simulink model "BBC_10"  (R2022b)
settings: Solver=VariableStepAuto  StartTime=0.0  StopTime=1.5  RelTol=1e-3
undefined symbols (not defined in the file): dEv, sigbuilder_block, X, Y
libraries: spsMosfetLib x4, spsSeriesRLCBranchLib x4, spsCurrentMeasurementLib x2, spsVoltageMeasurementLib x2, dspstat3 x1, simulink x1, spsGroundLib x1, spsControlledVoltageSourceLib x1, spspowerguiLib x1
settings Model: Creator=Dopechuro  LastModifiedBy=Dopechuro

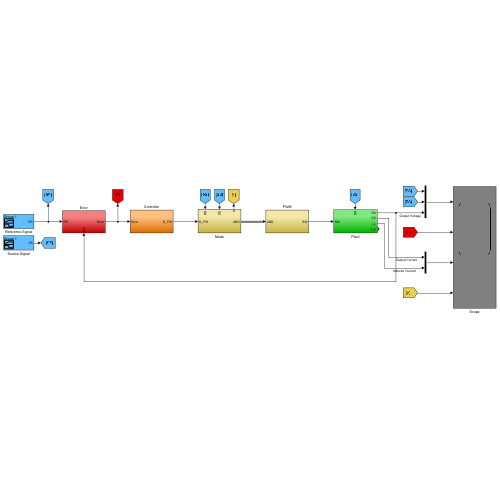
[thumbnail: Simulink's stored preview of the top-level diagram]
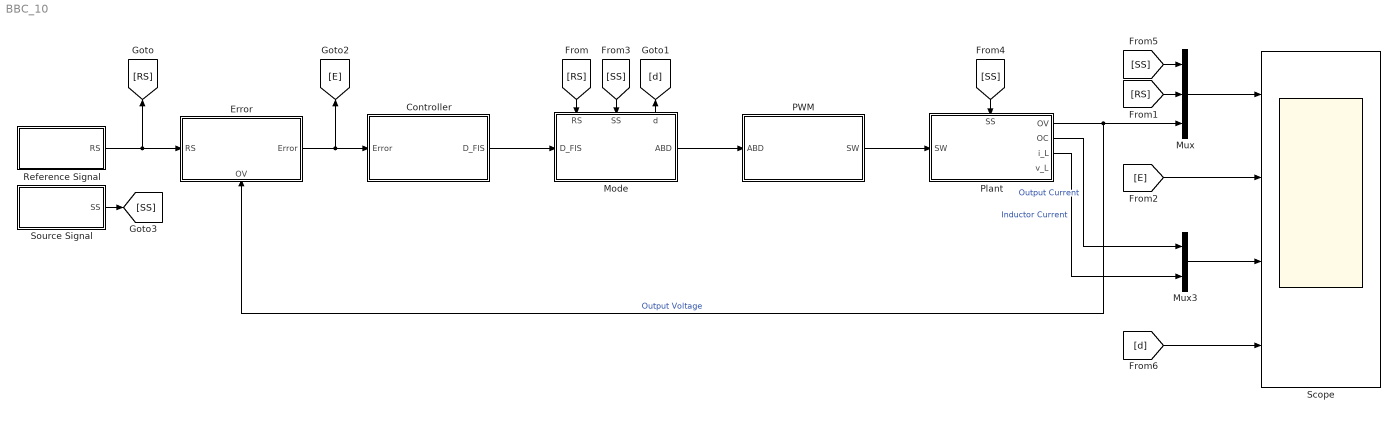
== system BBC_10 ==
  Controller : Subsystem
  Error : Subsystem
      settings: PortSchema="{\"entries\":[{\"content\":{\"sides\":[{\"content\":{\"connectorIds\":[\"In1\"]},\"type\":\"ConnectorPlacement.EquallySpacedRectSide\",\"uuid\":\"17a1441e-cc20-45c1-b94d-2797150f41f6\"},{\"content\":{\"connectorIds\":[\"Out1\"],\"side\":\"RIGHT\"},\"type\":\"ConnectorPlacement.EquallySpacedRectSide\",\"uuid\":\"0eaf207d-efc8-435f-a7b8-030690917f23\"},{\"content\":{\"connectorIds\":[],\"side\":\"TOP\"},\"type\":\"ConnectorPlacement.EquallySpacedRectSide\",\"uuid\":\"e36a2cea-826c-4841-9b9b-81d458cfbbc3\"},{\"content\":{\"connectorIds\":[\"In2\"],\"side\":\"BOTTOM\"},\"type\":\"ConnectorPlacement.EquallySpacedRectSide\",\"uuid\":\"071bf484-cc76-4d4d-9853-4ed74954b615\"}]},\"type\":\"ConnectorPlacement.EquallySpacedConnector\",\"uuid\":\"670cfee0-0ffb-439b-ae3a-e57aa259e987\"}],\"packageUris\":[\"http://schema.mathworks.com/mf0/Connector/R2020b\"],\"version\":\"1.0\"}"
  Mode : Subsystem
      settings: PortSchema="{\"entries\":[{\"content\":{\"sides\":[{\"content\":{\"connectorIds\":[\"In1\"]},\"type\":\"ConnectorPlacement.EquallySpacedRectSide\",\"uuid\":\"22e8c9bf-f581-4102-833a-b5611cc3792f\"},{\"content\":{\"connectorIds\":[\"Out1\"],\"side\":\"RIGHT\"},\"type\":\"ConnectorPlacement.EquallySpacedRectSide\",\"uuid\":\"f8140a0f-c6c9-4e51-870e-44c023f722d5\"},{\"content\":{\"connectorIds\":[\"In2\",\"In3\",\"Out2\"],\"side\":\"TOP\"},\"type\":\"ConnectorPlacement.EquallySpacedRectSide\",\"uuid\":\"10db0567-fbdd-40f4-a2fd-97d53c1d8902\"}]},\"type\":\"ConnectorPlacement.EquallySpacedConnector\",\"uuid\":\"7b381037-9dff-477f-a3a5-d3b1d369cb30\"}],\"packageUris\":[\"http://schema.mathworks.com/mf0/Connector/R2020b\"],\"version\":\"1.0\"}"
  Mux : Mux  Inputs=3
  Mux3 : Mux  Inputs=2
  PWM : Subsystem
  Plant : Subsystem
      settings: PortSchema="{\"entries\":[{\"content\":{\"sides\":[{\"content\":{\"connectorIds\":[\"In1\"]},\"type\":\"ConnectorPlacement.EquallySpacedRectSide\",\"uuid\":\"0ef50e83-df86-4363-90f2-24d802fe3b4b\"},{\"content\":{\"connectorIds\":[\"Out1\",\"Out2\",\"Out3\",\"Out4\"],\"side\":\"RIGHT\"},\"type\":\"ConnectorPlacement.EquallySpacedRectSide\",\"uuid\":\"773bb1cd-eb13-489f-85b5-8123b37f0dae\"},{\"content\":{\"connectorIds\":[\"In2\"],\"side\":\"TOP\"},\"type\":\"ConnectorPlacement.EquallySpacedRectSide\",\"uuid\":\"126728fb-74b0-43b7-8ac4-8c3020c4e5e7\"}]},\"type\":\"ConnectorPlacement.EquallySpacedConnector\",\"uuid\":\"c08fd5b4-960e-4ff5-bbd6-4b76aceb8bf8\"}],\"packageUris\":[\"http://schema.mathworks.com/mf0/Connector/R2020b\"],\"version\":\"1.0\"}"
  Reference Signal : Subsystem  Tag=STV Subsys  LoadFcn=sigbuilder_block('load');  StartFcn=sigbuilder_block('start');  StopFcn=sigbuilder_block('stop');  ClipboardFcn=sigbuilder_block('clipboard');  mask(Sigbuilder block){tuvar=[0:10]}
      mask help: Simulink:masks:SigbuilderBlock_MD
      mask init:
      | if ~strcmp(get_param(bdroot(gcbh),'SimulationStatus'),'stopped') tuvar = sigbuilder_block('maskInit'); end
      settings: CopyFcn=sigbuilder_block('copy');  DeleteFcn=sigbuilder_block('delete');  ModelCloseFcn=sigbuilder_block('modelClose');  PreSaveFcn=sigbuilder_block('preSave');  PauseFcn=sigbuilder_block('pause');  ContinueFcn=sigbuilder_block('continue');  NameChangeFcn=sigbuilder_block('namechange');  OpenFcn=sigbuilder_block('open',[0.75 0.75 958.5 1015.5 ]);  CloseFcn=sigbuilder_block('close');
      mask Display: plot(0, 0, 100, 100,[2, 2, 32, 32, 2], [68, 8, 8, 68, 68],[32, 2], [38, 38], [32, 19, 2],[53, 60, 44], [32, 17, 17, 2],[16, 16, 31, 31]);txt = getActiveGroup(gcbh);text(2, 100, txt,'verticalAlignment', 'top');
  Scope : Scope  NumInputPorts=4
  Source Signal : Subsystem  Tag=STV Subsys  LoadFcn=sigbuilder_block('load');  StartFcn=sigbuilder_block('start');  StopFcn=sigbuilder_block('stop');  ClipboardFcn=sigbuilder_block('clipboard');  mask(Sigbuilder block){tuvar=[0:10]}
      mask help: Simulink:masks:SigbuilderBlock_MD
      mask init:
      | if ~strcmp(get_param(bdroot(gcbh),'SimulationStatus'),'stopped') tuvar = sigbuilder_block('maskInit'); end
      settings: CopyFcn=sigbuilder_block('copy');  DeleteFcn=sigbuilder_block('delete');  ModelCloseFcn=sigbuilder_block('modelClose');  PreSaveFcn=sigbuilder_block('preSave');  PauseFcn=sigbuilder_block('pause');  ContinueFcn=sigbuilder_block('continue');  NameChangeFcn=sigbuilder_block('namechange');  OpenFcn=sigbuilder_block('open',[0.75 0.75 958.5 1015.5 ]);  CloseFcn=sigbuilder_block('close');
      mask Display: plot(0, 0, 100, 100,[2, 2, 32, 32, 2], [68, 8, 8, 68, 68],[32, 2], [38, 38], [32, 19, 2],[53, 60, 44], [32, 17, 17, 2],[16, 16, 31, 31]);txt = getActiveGroup(gcbh);text(2, 100, txt,'verticalAlignment', 'top');
  wires:
  Mux3/1 -> Scope/3
  Error/1(Error) -> [E], Controller/1(Error)
  [E] -> Scope/2
  [RS] -> Mux/2
  Reference Signal/1(RS) -> [RS], Error/1(RS)
  Source Signal/1(SS) -> [SS]
  [RS] -> Mode/2(RS)
  [SS] -> Mode/3(SS)
  Mode/2(d) -> [d]
  [SS] -> Mux/1
  [d] -> Scope/4
  Mode/1(ABD) -> PWM/1(ABD)
  PWM/1(SW) -> Plant/1(SW)
  Plant/1(OV) -> Mux/3, Error/2(OV)  "Output Voltage"
  [SS] -> Plant/2(SS)
  Plant/2(OC) -> Mux3/1  "Output Current"
  Plant/3(i_L) -> Mux3/2  "Inductor Current"
  Controller/1(D_FIS) -> Mode/1(D_FIS)
  Mux/1 -> Scope/1

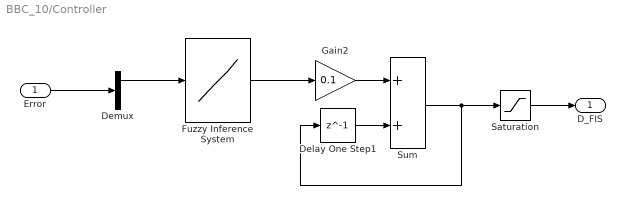
== system BBC_10/Controller ==
  Error : Inport
  Delay One Step1 : Delay  DelayLength=1
  Demux : Demux  Outputs=2
  Fuzzy Inference System : Lookup_n-D  NumberOfTableDimensions=1  LookupTableObject=''  BreakpointsForDimension1=X  BreakpointsForDimension2=dEv  BreakpointsForDimension1FirstPoint=10  BreakpointsForDimension2FirstPoint=10  BreakpointsForDimension1Spacing=12  BreakpointsForDimension2Spacing=12  IndexSearchMethod=Evenly spaced points  Table=Y  InterpMethod=Nearest  DiagnosticForOutOfRangeInput=Warning  InternalRulePriority=Speed  OutDataTypeStr=Inherit: Inherit from 'Table data'  RndMeth=Simplest
  Gain2 : Gain  Gain=0.1
  Saturation : Saturate
  Sum : Sum
  D_FIS : Outport
  wires:
  Delay One Step1/1 -> Sum/2
  Sum/1 -> Saturation/1, Delay One Step1/1
  Gain2/1 -> Sum/1
  Fuzzy Inference System/1 -> Gain2/1
  Saturation/1 -> D_FIS/1
  Error/1 -> Demux/1
  Demux/1 -> Fuzzy Inference System/1

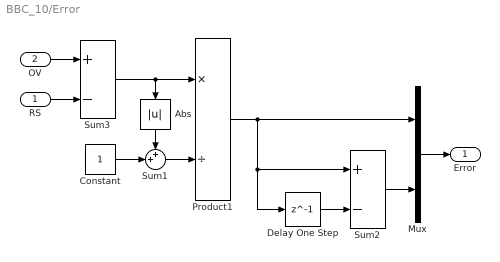
== system BBC_10/Error ==
  RS : Inport  SampleTime=1e-3
  OV : Inport  Port=2  SampleTime=1e-3
  Abs : Abs  SaturateOnIntegerOverflow=off
  Constant : Constant
  Delay One Step : Delay  DelayLength=1
  Mux : Mux  Inputs=2
  Product1 : Product  Inputs=*/
  Sum1 : Sum  Inputs=++|
  Sum2 : Sum  Inputs=+-
  Sum3 : Sum  Inputs=+-
  Error : Outport
  wires:
  Delay One Step/1 -> Sum2/2
  RS/1 -> Sum3/2
  Sum3/1 -> Abs/1, Product1/1
  Sum1/1 -> Product1/2
  Constant/1 -> Sum1/2
  Product1/1 -> Delay One Step/1, Sum2/1, Mux/1
  Abs/1 -> Sum1/1
  Sum2/1 -> Mux/2
  Mux/1 -> Error/1
  OV/1 -> Sum3/1

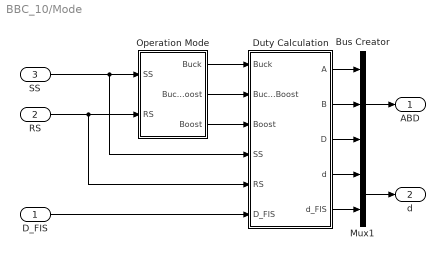
== system BBC_10/Mode ==
  D_FIS : Inport
  RS : Inport  Port=2  SampleTime=1e-3
  SS : Inport  Port=3  SampleTime=1e-3
  Bus Creator : BusCreator  Inputs=3
  Duty Calculation : Subsystem
  Mux1 : Mux  Inputs=2
  Operation Mode : Subsystem
  ABD : Outport
  d : Outport  Port=2
  wires:
  Operation Mode/2(Buck-Boost) -> Duty Calculation/2(Buck-Boost)
  SS/1 -> Operation Mode/1(SS), Duty Calculation/4(SS)
  RS/1 -> Operation Mode/2(RS), Duty Calculation/5(RS)
  Operation Mode/1(Buck) -> Duty Calculation/1(Buck)
  Operation Mode/3(Boost) -> Duty Calculation/3(Boost)
  D_FIS/1 -> Duty Calculation/6(D_FIS)
  Duty Calculation/5(d_FIS) -> Mux1/2
  Duty Calculation/4(d) -> Mux1/1
  Mux1/1 -> d/1
  Duty Calculation/1(A) -> Bus Creator/1
  Duty Calculation/2(B) -> Bus Creator/2
  Duty Calculation/3(D) -> Bus Creator/3
  Bus Creator/1 -> ABD/1

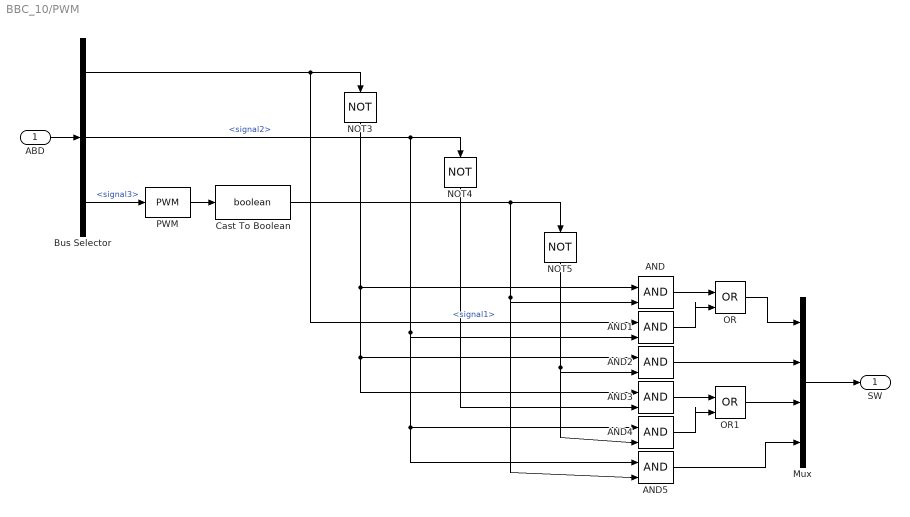
== system BBC_10/PWM ==
  ABD : Inport
  AND{,1..5} (6 alike) : Logic  IconShape=distinctive  AllPortsSameDT=off  OutDataTypeStr=boolean
  Bus Selector : BusSelector  OutputSignals=signal1,signal2,signal3
  Cast To Boolean : DataTypeConversion  OutDataTypeStr=boolean  SaturateOnIntegerOverflow=off  RndMeth=Floor
  Mux : Mux
  NOT3 : Logic  Operator=NOT  IconShape=distinctive  AllPortsSameDT=off  OutDataTypeStr=boolean
  NOT4 : Logic  Operator=NOT  IconShape=distinctive  AllPortsSameDT=off  OutDataTypeStr=boolean
  NOT5 : Logic  Operator=NOT  IconShape=distinctive  AllPortsSameDT=off  OutDataTypeStr=boolean
  OR : Logic  Operator=OR  IconShape=distinctive  AllPortsSameDT=off  OutDataTypeStr=boolean
  OR1 : Logic  Operator=OR  IconShape=distinctive  AllPortsSameDT=off  OutDataTypeStr=boolean
  PWM : simulink/Discontinuities/PWM  DisableCoverage=on  Period=1e-5  InitialDelay=0  DisallowZeroDutyCycle=off  RunAtFixedTimeIntervals=off  SampleTime=0.1
  SW : Outport
  wires:
  NOT5/1 -> AND4/2, AND2/2
  Bus Selector/2 -> AND1/2, AND4/1, AND5/1, NOT4/1  "<signal2>"
  Bus Selector/1 -> NOT3/1, AND1/1  "<signal1>"
  Cast To Boolean/1 -> NOT5/1, AND5/2, AND/2
  NOT3/1 -> AND/1, AND2/1, AND3/1
  AND1/1 -> OR/2
  NOT4/1 -> AND3/2
  AND4/1 -> OR1/2
  AND/1 -> OR/1
  AND3/1 -> OR1/1
  OR/1 -> Mux/1
  PWM/1 -> Cast To Boolean/1
  Mux/1 -> SW/1
  AND2/1 -> Mux/2
  OR1/1 -> Mux/3
  AND5/1 -> Mux/4
  Bus Selector/3 -> PWM/1  "<signal3>"
  ABD/1 -> Bus Selector/1

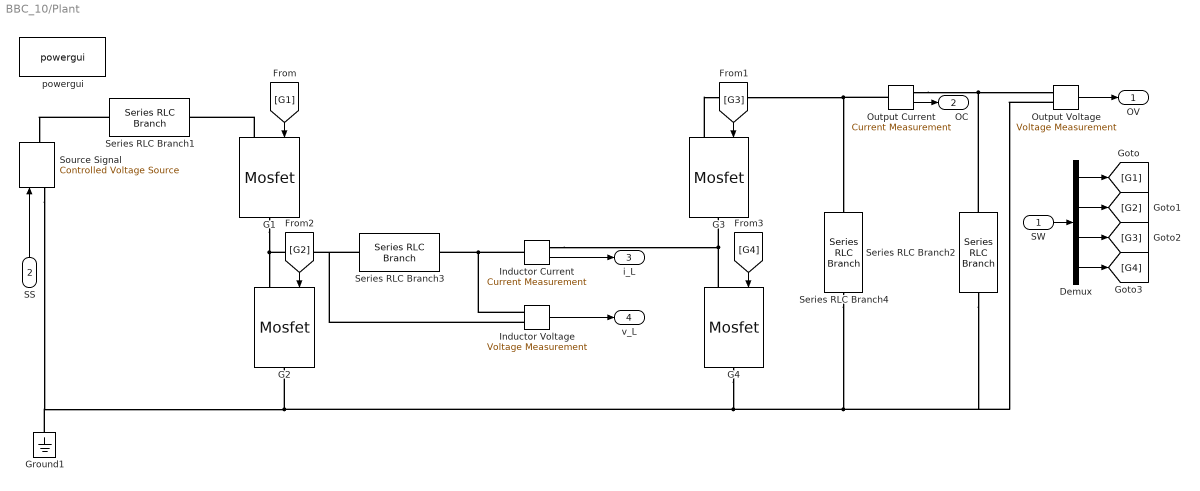
== system BBC_10/Plant ==
  SW : Inport
  SS : Inport  Port=2
  Demux : Demux
  G{1..4} (4 alike) : spsMosfetLib/Mosfet  Ron=0.1  Lon=0  Rd=0.01  Vfd=0  IC=0  Rs=1e5  Cs=inf  Measurements=off
  Ground1 : spsGroundLib/Ground  LConnTagsString=a
  Inductor Current : spsCurrentMeasurementLib/Current Measurement  PhasorSimulation=off  OutputType=Complex  PSBequivalent=0
  Inductor Voltage : spsVoltageMeasurementLib/Voltage Measurement  PhasorSimulation=off  OutputType=Complex  PSBequivalent=0
  Output Current : spsCurrentMeasurementLib/Current Measurement  PhasorSimulation=off  OutputType=Complex  PSBequivalent=0
  Output Voltage : spsVoltageMeasurementLib/Voltage Measurement  PhasorSimulation=off  OutputType=Complex  PSBequivalent=0
  Series RLC Branch1 : spsSeriesRLCBranchLib/Series RLC Branch  LConnTagsString=__new0  RConnTagsString=__new0  BranchType=R  Resistance=0.1  Inductance=1e-3  SetiL0=off  InitialCurrent=0  Capacitance=1e-6  Setx0=off  InitialVoltage=0  Measurements=None
  Series RLC Branch2 : spsSeriesRLCBranchLib/Series RLC Branch  LConnTagsString=__new0  RConnTagsString=__new0  BranchType=R  Resistance=24  Inductance=1e-3  SetiL0=off  InitialCurrent=0  Capacitance=1000e-6  Setx0=off  InitialVoltage=0  Measurements=None
  Series RLC Branch3 : spsSeriesRLCBranchLib/Series RLC Branch  LConnTagsString=__new0  RConnTagsString=__new0  BranchType=RL  Resistance=0.1  Inductance=0.434e-3  SetiL0=off  InitialCurrent=0  Capacitance=1e-6  Setx0=off  InitialVoltage=0  Measurements=None
  Series RLC Branch4 : spsSeriesRLCBranchLib/Series RLC Branch  LConnTagsString=__new0  RConnTagsString=__new0  BranchType=RC  Resistance=0.01  Inductance=1e-3  SetiL0=off  InitialCurrent=0  Capacitance=9.143e-6  Setx0=off  InitialVoltage=0  Measurements=None
  Source Signal : spsControlledVoltageSourceLib/Controlled Voltage Source  Initialize=off  Source_Type=DC  Amplitude=0  Phase=0  Frequency=0  Measurements=None
  powergui : spspowerguiLib/powergui  Priority=1  SimulationMode=Continuous  SampleTime=1e-6  frequency=60  Iterations=50  frequencyindice=0  Pbase=100e6  ErrMax=1e-4  UnitsV=kV  UnitsW=MW  buscounter=0  FunctionMessages=off  echomessages=off  EnableUseOfTLC=off  CurrentSourceSwitches=off  DisableSnubberDevices=off  DisableRonSwitches=off  DisableVfSwitches=off  DisplayEquations=off  AutomaticDiscreteSolvers=off  SolverType=Tustin/Backward Euler (TBE)  Interpol=off  ExternalGateDelay=off  methode=off  Ts=100  x0status=blocks  SPID=on  SwTol=0  HookPort=off  NonlinearTolerance=1e-4  nMaxIteration=100  ContinueOnMaxIteration=off  RestoreLinks=warning  ResistiveCurrentMeasurement=off  Frange=[0:2:500]  Ylog=off  Xlog=on  ShowGrid=off  save=off  variable=ZData  structure=0  ZoomFFT=off  StartTime=0.0  cycles=1  DisplayStyle=1  fundamental=60  FreqAxis=off  MaxFrequency=1000  frequencyindicesteady=1  RmsSteady=1  display=off
  OV : Outport
  OC : Outport  Port=2
  i_L : Outport  Port=3
  v_L : Outport  Port=4
  wires:
  SS/1 -> Source Signal/1
  Inductor Current/1 -> i_L/1
  Output Voltage/1 -> OV/1
  Inductor Voltage/1 -> v_L/1
  Output Current/1 -> OC/1
  [G2] -> G2/1
  [G1] -> G1/1
  [G3] -> G3/1
  [G4] -> G4/1
  Demux/1 -> [G1]
  Demux/2 -> [G2]
  Demux/3 -> [G3]
  Demux/4 -> [G4]
  SW/1 -> Demux/1
  connections:
  G1/LConn1 -- Series RLC Branch1/RConn1
  Inductor Current/LConn1 -- Inductor Voltage/LConn2 -- Series RLC Branch3/RConn1
  G4/LConn1 -- Inductor Current/RConn1 -- G3/RConn1
  G4/RConn1 -- Output Voltage/LConn2 -- Series RLC Branch2/RConn1 -- Series RLC Branch4/RConn1 -- Source Signal/LConn1 -- Ground1/LConn1 -- G2/RConn1
  G1/RConn1 -- Inductor Voltage/LConn1 -- Series RLC Branch3/LConn1 -- G2/LConn1
  Series RLC Branch1/LConn1 -- Source Signal/RConn1
  Output Current/RConn1 -- Output Voltage/LConn1 -- Series RLC Branch2/LConn1
  G3/LConn1 -- Output Current/LConn1 -- Series RLC Branch4/LConn1

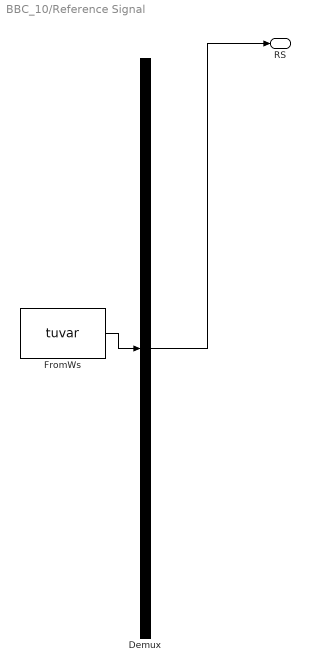
== system BBC_10/Reference Signal ==
  Demux : Demux  Tag=STV Demux  Outputs=1
      settings: DisplayOption=none
  FromWs : FromWorkspace  Tag=STV FromWs  VariableName=tuvar
      SigBuilderData=|
      | common.afterFinalStr = 'Extrapolate'
      | common.sampleTime = 0
      | dataSet.timeRange = [0 3]
      | dataSet.name = 'Group 1'
      | sbobj.Groups.Name = 'Group 1'
      | sbobj.Groups.Signals.Name = 'RS'
      | sbobj.Groups.Signals.XData = [0 3]
      | sbobj.Groups.Signals.YData = [48 48]
      | sbobj.Groups.TimeRange = [0 3]
  RS : Outport  Tag=STV Outport
  wires:
  FromWs/1 -> Demux/1
  Demux/1 -> RS/1

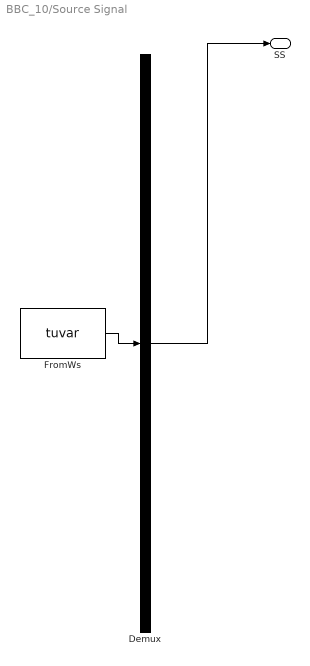
== system BBC_10/Source Signal ==
  Demux : Demux  Tag=STV Demux  Outputs=1
      settings: DisplayOption=none
  FromWs : FromWorkspace  Tag=STV FromWs  VariableName=tuvar
      SigBuilderData=|
      | common.afterFinalStr = 'Extrapolate'
      | common.sampleTime = 0
      | dataSet.timeRange = [0 3]
      | dataSet.name = 'Group 1'
      | sbobj.Groups.Name = 'Group 1'
      | sbobj.Groups.Signals.Name = 'SS'
      | sbobj.Groups.Signals.XData = [0 3]
      | sbobj.Groups.Signals.YData = [70 35]
      | sbobj.Groups.TimeRange = [0 3]
  SS : Outport  Tag=STV Outport
  wires:
  FromWs/1 -> Demux/1
  Demux/1 -> SS/1

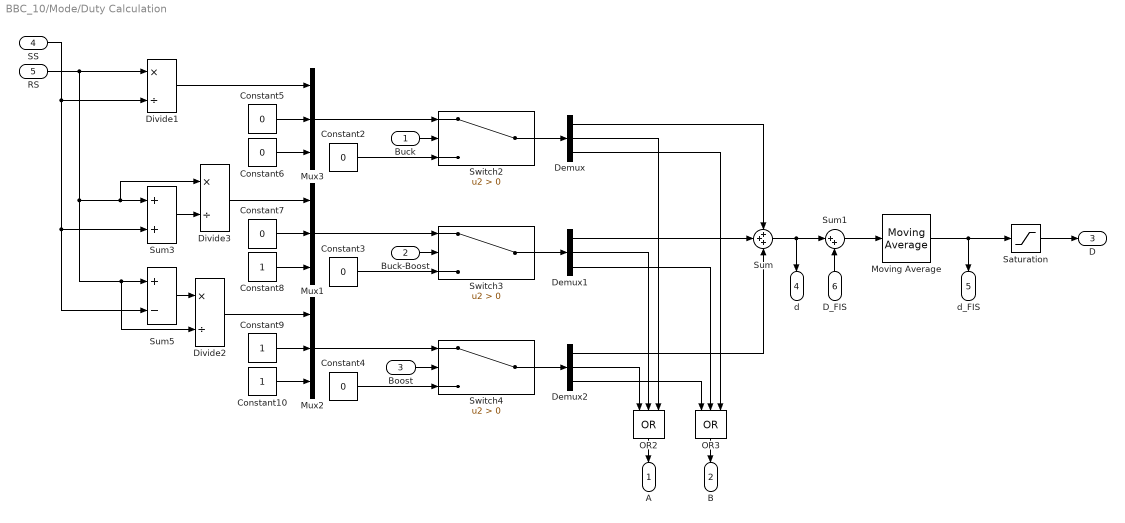
== system BBC_10/Mode/Duty Calculation ==
  Buck : Inport
  Buck-Boost : Inport  Port=2
  Boost : Inport  Port=3
  SS : Inport  Port=4
  RS : Inport  Port=5
  D_FIS : Inport  Port=6
  Constant10 : Constant
  Constant{2..7} (6 alike) : Constant  Value=0
  Constant8 : Constant
  Constant9 : Constant
  Demux : Demux  Outputs=3
  Demux1 : Demux  Outputs=3
  Demux2 : Demux  Outputs=3
  Divide1 : Product  Inputs=*/
  Divide2 : Product  Inputs=*/
  Divide3 : Product  Inputs=*/
  Moving Average : dspstat3/Moving Average  Method=Exponential weighting  ForgettingFactorPort=off  SpecifyWindowLength=on  WindowLength=4  OverlapLength=3  AllowArbitraryInputLength=off  ForgettingFactor=0.9  SimulateUsing=Code generation
  Mux1 : Mux  Inputs=3
  Mux2 : Mux  Inputs=3
  Mux3 : Mux  Inputs=3
  OR2 : Logic  Operator=OR  Inputs=3  IconShape=distinctive  AllPortsSameDT=off  OutDataTypeStr=boolean
  OR3 : Logic  Operator=OR  Inputs=3  IconShape=distinctive  AllPortsSameDT=off  OutDataTypeStr=boolean
  Saturation : Saturate  UpperLimit=0.8  LowerLimit=0.2
  Sum : Sum  Inputs=+++
  Sum1 : Sum  Inputs=|++
  Sum3 : Sum
  Sum5 : Sum  Inputs=+-
  Switch2 : Switch  Criteria=u2 > Threshold  SaturateOnIntegerOverflow=off  InputSameDT=off
  Switch3 : Switch  Criteria=u2 > Threshold  SaturateOnIntegerOverflow=off  InputSameDT=off
  Switch4 : Switch  Criteria=u2 > Threshold  SaturateOnIntegerOverflow=off  InputSameDT=off
  A : Outport
  B : Outport  Port=2
  D : Outport  Port=3
  d : Outport  Port=4
  d_FIS : Outport  Port=5
  wires:
  Constant6/1 -> Mux3/3
  Constant2/1 -> Switch2/3
  Switch4/1 -> Demux2/1
  Sum3/1 -> Divide3/2
  Constant5/1 -> Mux3/2
  Mux3/1 -> Switch2/1
  Constant8/1 -> Mux1/3
  Demux1/1 -> Sum/2
  D_FIS/1 -> Sum1/2
  Switch3/1 -> Demux1/1
  Switch2/1 -> Demux/1
  Constant4/1 -> Switch4/3
  Demux/3 -> OR3/3
  Buck-Boost/1 -> Switch3/2
  Demux2/1 -> Sum/3
  Demux2/2 -> OR2/1
  Sum5/1 -> Divide2/1
  RS/1 -> Divide1/1, Sum3/1, Divide3/1, Sum5/1, Divide2/2
  Divide1/1 -> Mux3/1
  Demux/2 -> OR2/3
  Demux2/3 -> OR3/1
  Saturation/1 -> D/1
  Demux1/2 -> OR2/2
  Constant10/1 -> Mux2/3
  Demux/1 -> Sum/1
  OR3/1 -> B/1
  Mux2/1 -> Switch4/1
  Demux1/3 -> OR3/2
  Constant3/1 -> Switch3/3
  SS/1 -> Divide1/2, Sum3/2, Sum5/2
  Divide2/1 -> Mux2/1
  Mux1/1 -> Switch3/1
  Constant9/1 -> Mux2/2
  Constant7/1 -> Mux1/2
  Divide3/1 -> Mux1/1
  OR2/1 -> A/1
  Boost/1 -> Switch4/2
  Buck/1 -> Switch2/2
  Sum1/1 -> Moving Average/1
  Sum/1 -> Sum1/1, d/1
  Moving Average/1 -> Saturation/1, d_FIS/1

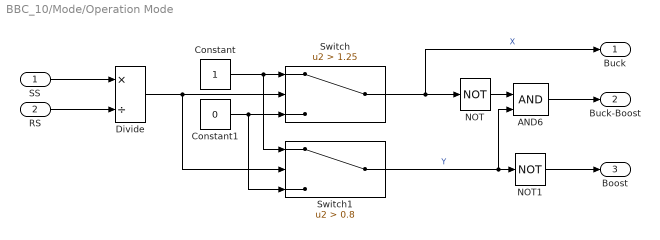
== system BBC_10/Mode/Operation Mode ==
  SS : Inport
  RS : Inport  Port=2
  AND6 : Logic  IconShape=distinctive  AllPortsSameDT=off  OutDataTypeStr=boolean
  Constant : Constant
  Constant1 : Constant  Value=0
  Divide : Product  Inputs=*/
  NOT : Logic  Operator=NOT  IconShape=distinctive  AllPortsSameDT=off  OutDataTypeStr=boolean
  NOT1 : Logic  Operator=NOT  IconShape=distinctive  AllPortsSameDT=off  OutDataTypeStr=boolean
  Switch : Switch  Criteria=u2 > Threshold  Threshold=1.25  SaturateOnIntegerOverflow=off  InputSameDT=off
  Switch1 : Switch  Criteria=u2 > Threshold  Threshold=0.8  SaturateOnIntegerOverflow=off  InputSameDT=off
  Buck : Outport
  Buck-Boost : Outport  Port=2
  Boost : Outport  Port=3
  wires:
  RS/1 -> Divide/2
  Constant/1 -> Switch1/1, Switch/1
  Divide/1 -> Switch1/2, Switch/2
  NOT/1 -> AND6/1
  Constant1/1 -> Switch1/3, Switch/3
  SS/1 -> Divide/1
  AND6/1 -> Buck-Boost/1
  NOT1/1 -> Boost/1
  Switch1/1 -> NOT1/1, AND6/2  "Y"
  Switch/1 -> Buck/1, NOT/1  "X"
